simulink model "EulerSolver_Master_20161229"  (R2016a)
settings: Solver=ode45  StartTime=0.0  StopTime=20  MaxStep=0.001  RelTol=1e-5  AbsTol=1e-5
values from neighbouring files (symbols this model uses):
  I = [3 3 7]    [EulerSolverVariables_Master_20161229.m]
  N = [0 0 0]    [EulerSolverVariables_Master_20161229.m]
  w = [0 0 5]    [EulerSolverVariables_Master_20161229.m]
settings Model: Creator=Kevin  LastModifiedBy=Kevin
settings GRTTargetCC: GeneratePreprocessorConditionals=Use local settings
settings SimscapeCC: SimscapeLogType=all  SimscapeLogDataHistory=10000

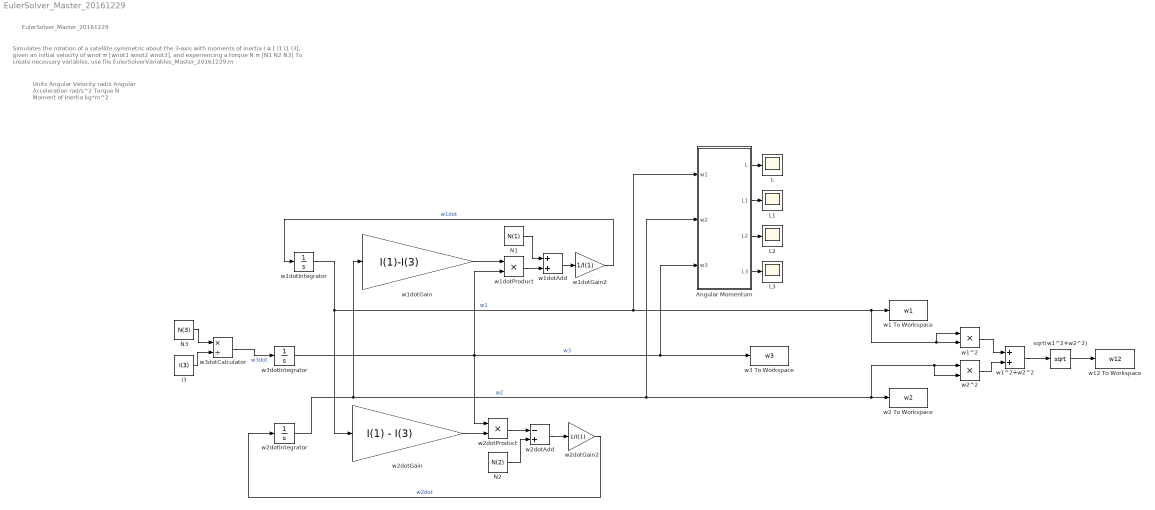
== system EulerSolver_Master_20161229 ==
  note: Units
      | Angular Velocity rad/s
      | Angular Acceleration rad/s^2
      | Torque N
      | Moment of Inertia kg*m^2
  note: Simulates the rotation of a satellite symmetric about the 3-axis with moments of inertia I = [ I1 I1 I3], given an initial velocity of wnot = [wnot1 wnot2 wnot3], and experiencing a torque N = [N1 N2 N3]
      | To create necessary variables, use file EulerSolverVariables_Master_20161229.m
  note: EulerSolver_Master_20161229
  Angular Momentum : Subsystem
  I3 : Constant  Value=I(3)
  L{,1..3} (4 alike) : Scope
  N1 : Constant  Value=N(1)
  N2 : Constant  Value=N(2)
  N3 : Constant  Value=N(3)
  sqrt(w1^2+w2^2) : Sqrt  SaturateOnIntegerOverflow=on
  w1 To Workspace : ToWorkspace  VariableName=w1  SaveFormat=Timeseries  SampleTime=-1
  w12 To Workspace : ToWorkspace  VariableName=w12  SaveFormat=Timeseries  SampleTime=-1
  w1^2 : Product
  w1^2+w2^2 : Sum
  w1dotAdd : Sum
  w1dotGain : Gain  Gain=I(1)-I(3)
  w1dotGain2 : Gain  Gain=1/I(1)
  w1dotIntegrator : Integrator  InitialCondition=w(1)
  w1dotProduct : Product
  w2 To Workspace : ToWorkspace  VariableName=w2  SaveFormat=Timeseries  SampleTime=-1
  w2^2 : Product
  w2dotAdd : Sum  Inputs=-+
  w2dotGain : Gain  Gain=I(1) - I(3)
  w2dotGain2 : Gain  Gain=1/I(1)
  w2dotIntegrator : Integrator  InitialCondition=w(2)
  w2dotProduct : Product
  w3 To Workspace : ToWorkspace  VariableName=w3  SaveFormat=Timeseries  SampleTime=-1
  w3dotCalculator : Product  Inputs=*/
  w3dotIntegrator : Integrator  InitialCondition=w(3)
  wires:
  w1dotGain2/1 -> w1dotIntegrator/1  "w1dot"
  w1dotIntegrator/1 -> w2dotGain/1, Angular Momentum/1(w1), w1 To Workspace/1, w1^2/2, w1^2/1  "w1"
  w1dotAdd/1 -> w1dotGain2/1
  w2dotAdd/1 -> w2dotGain2/1
  w2dotGain2/1 -> w2dotIntegrator/1  "w2dot"
  N2/1 -> w2dotAdd/2
  N1/1 -> w1dotAdd/1
  w3dotCalculator/1 -> w3dotIntegrator/1  "w3dot"
  w1dotGain/1 -> w1dotProduct/1
  w2dotGain/1 -> w2dotProduct/2
  w3dotIntegrator/1 -> w2dotProduct/1, w1dotProduct/2, w3 To Workspace/1, Angular Momentum/3(w3)  "w3"
  w2dotProduct/1 -> w2dotAdd/1
  w1dotProduct/1 -> w1dotAdd/2
  w2dotIntegrator/1 -> w2 To Workspace/1, w2^2/2, w2^2/1, Angular Momentum/2(w2), w1dotGain/1  "w2"
  w2^2/1 -> w1^2+w2^2/2
  w1^2/1 -> w1^2+w2^2/1
  sqrt(w1^2+w2^2)/1 -> w12 To Workspace/1
  w1^2+w2^2/1 -> sqrt(w1^2+w2^2)/1
  Angular Momentum/1(L) -> L/1
  Angular Momentum/2(L1) -> L1/1
  Angular Momentum/3(L2) -> L2/1
  Angular Momentum/4(L3) -> L3/1
  N3/1 -> w3dotCalculator/1
  I3/1 -> w3dotCalculator/2

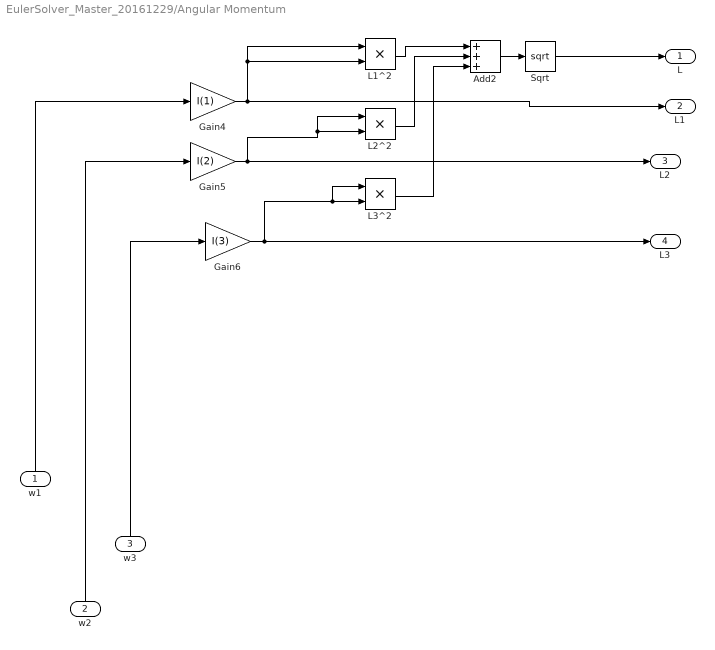
== system EulerSolver_Master_20161229/Angular Momentum ==
  w1 : Inport
  w2 : Inport  Port=2
  w3 : Inport  Port=3
  Add2 : Sum  Inputs=+++
  Gain4 : Gain  Gain=I(1)
  Gain5 : Gain  Gain=I(2)
  Gain6 : Gain  Gain=I(3)
  L1^2 : Product
  L2^2 : Product
  L3^2 : Product
  Sqrt : Sqrt  SaturateOnIntegerOverflow=on
  L : Outport
  L1 : Outport  Port=2
  L2 : Outport  Port=3
  L3 : Outport  Port=4
  wires:
  Gain5/1 -> L2/1, L2^2/2, L2^2/1
  L1^2/1 -> Add2/1
  Sqrt/1 -> L/1
  L3^2/1 -> Add2/3
  Add2/1 -> Sqrt/1
  L2^2/1 -> Add2/2
  Gain6/1 -> L3/1, L3^2/2, L3^2/1
  Gain4/1 -> L1/1, L1^2/2, L1^2/1
  w3/1 -> Gain6/1
  w2/1 -> Gain5/1
  w1/1 -> Gain4/1
